simulink library "ARBI_lib"  (Simulink 7.5)
settings: Solver=ode45  StartTime=0.0  StopTime=10.0  RelTol=1e-3
values from neighbouring files (symbols this model uses):
  pARBI_st_AirbagError_C = Simulink.Parameter    [ARBI_par.m]
  pARBI_st_Crash_C = Simulink.Parameter    [ARBI_par.m]
libraries: BaseOperationLib_Browser x6, PES_CZ_FAW x2, simulink x2
settings Model: Creator=wuaibin  LastModifiedBy=wuaibin

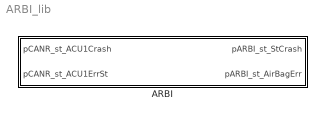
== system ARBI_lib ==
  ARBI : Subsystem  TreatAsAtomicUnit=on

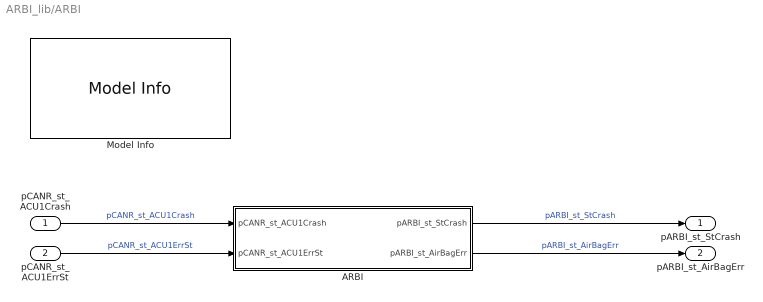
== system ARBI_lib/ARBI ==
  pCANR_st_ACU1Crash : Inport  OutDataType=fixdt(1, 16)  OutScaling=2^0
  pCANR_st_ACU1ErrSt : Inport  Port=2  OutDataType=fixdt(1, 16)  OutScaling=2^0
  ARBI : Subsystem  TreatAsAtomicUnit=on
  Model Info : simulink/Model-Wide Utilities/Model Info  SystemSampleTime=-1  InitialBlockCM=None  BlockCM=None  Frame=on  DisplayStringWithTags=Model Info\nCreated: %<Created>\nCreator: zhangqiang  HorizontalTextAlignment=Center  LeftAlignmentValue=0.5  SourceBlockDiagram=untitled  TagMaxNumber=20
  pARBI_st_StCrash : Outport  OutDataType=fixdt(1, 16)  OutScaling=2^0
  pARBI_st_AirBagErr : Outport  Port=2  OutDataType=fixdt(1, 16)  OutScaling=2^0
  wires:
  ARBI/1(pARBI_st_StCrash) -> pARBI_st_StCrash/1  "pARBI_st_StCrash"
  pCANR_st_ACU1Crash/1 -> ARBI/1(pCANR_st_ACU1Crash)  "pCANR_st_ACU1Crash"
  pCANR_st_ACU1ErrSt/1 -> ARBI/2(pCANR_st_ACU1ErrSt)  "pCANR_st_ACU1ErrSt"
  ARBI/2(pARBI_st_AirBagErr) -> pARBI_st_AirBagErr/1  "pARBI_st_AirBagErr"

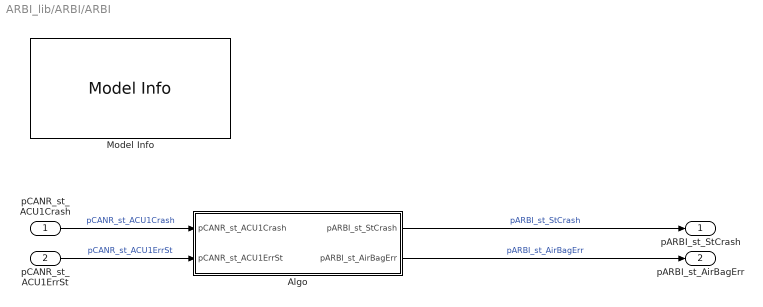
== system ARBI_lib/ARBI/ARBI ==
  pCANR_st_ACU1Crash : Inport  OutDataType=fixdt(1, 16)  OutScaling=2^0
  pCANR_st_ACU1ErrSt : Inport  Port=2  OutDataType=fixdt(1, 16)  OutScaling=2^0
  Algo : Subsystem
  Model Info : simulink/Model-Wide Utilities/Model Info  SystemSampleTime=-1  InitialBlockCM=None  BlockCM=None  Frame=on  DisplayStringWithTags=Model Info\nCreated: %<Created>\nCreator: %<Creator>  HorizontalTextAlignment=Center  LeftAlignmentValue=0.5  SourceBlockDiagram=HQEV_HCU  TagMaxNumber=20
  pARBI_st_StCrash : Outport  OutDataType=fixdt(1, 16)  OutScaling=2^0
  pARBI_st_AirBagErr : Outport  Port=2  OutDataType=fixdt(1, 16)  OutScaling=2^0
  wires:
  Algo/2(pARBI_st_AirBagErr) -> pARBI_st_AirBagErr/1  "pARBI_st_AirBagErr"
  pCANR_st_ACU1ErrSt/1 -> Algo/2(pCANR_st_ACU1ErrSt)  "pCANR_st_ACU1ErrSt"
  pCANR_st_ACU1Crash/1 -> Algo/1(pCANR_st_ACU1Crash)  "pCANR_st_ACU1Crash"
  Algo/1(pARBI_st_StCrash) -> pARBI_st_StCrash/1  "pARBI_st_StCrash"

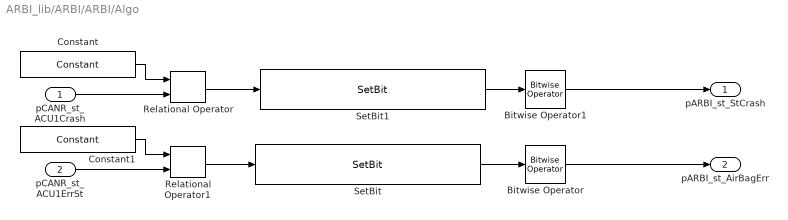
== system ARBI_lib/ARBI/ARBI/Algo ==
  pCANR_st_ACU1Crash : Inport  OutDataType=fixdt(1, 16)  OutScaling=2^0
  pCANR_st_ACU1ErrSt : Inport  Port=2  OutDataType=fixdt(1, 16)  OutScaling=2^0
  Bitwise Operator : BaseOperationLib_Browser/Others Unchanged/Bitwise Operator  logicop=OR  UseBitMask=off  BitMask=bin2dec('11011001')  BitMaskRealWorld=Stored Integer
  Bitwise Operator1 : BaseOperationLib_Browser/Others Unchanged/Bitwise Operator  logicop=OR  UseBitMask=off  BitMask=bin2dec('11011001')  BitMaskRealWorld=Stored Integer
  Constant : BaseOperationLib_Browser/Sources&Sinks/Constant  Value=pARBI_st_Crash_C  OutMin=[]  OutMax=[]  OutDataType=fixdt(1, 16)  ConRadixGroup=Use specified scaling  OutScaling=2^0  OutDataTypeStr=Inherit: Inherit from 'Constant value'
  Constant1 : BaseOperationLib_Browser/Sources&Sinks/Constant  Value=pARBI_st_AirbagError_C  OutMin=[]  OutMax=[]  OutDataType=fixdt(1, 16)  ConRadixGroup=Use specified scaling  OutScaling=2^0  OutDataTypeStr=Inherit: Inherit from 'Constant value'
  Relational Operator : BaseOperationLib_Browser/Logic Operations Changed/Relational Operator  Operator===  InputSameDT=on  LogicOutDataTypeMode=Specify via dialog  LogicDataType=PDT_Bool  OutDataTypeStr=PDT_Bool
  Relational Operator1 : BaseOperationLib_Browser/Logic Operations Changed/Relational Operator  Operator===  InputSameDT=on  LogicOutDataTypeMode=Specify via dialog  LogicDataType=PDT_Bool  OutDataTypeStr=PDT_Bool
  SetBit : PES_CZ_FAW/Discontinuities/SetBit  SystemSampleTime=-1  maska=FAWAirBagErrTyp.AIRBAG_ERROR
  SetBit1 : PES_CZ_FAW/Discontinuities/SetBit  SystemSampleTime=-1  maska=StaCrashTyp.CRASH
  pARBI_st_StCrash : Outport  OutDataType=fixdt(1, 16)  OutScaling=2^0
  pARBI_st_AirBagErr : Outport  Port=2  OutDataType=fixdt(1, 16)  OutScaling=2^0
  wires:
  SetBit1/1 -> Bitwise Operator1/1
  Bitwise Operator/1 -> pARBI_st_AirBagErr/1
  SetBit/1 -> Bitwise Operator/1
  Bitwise Operator1/1 -> pARBI_st_StCrash/1
  Relational Operator/1 -> SetBit1/1
  Relational Operator1/1 -> SetBit/1
  pCANR_st_ACU1ErrSt/1 -> Relational Operator1/2
  pCANR_st_ACU1Crash/1 -> Relational Operator/2
  Constant/1 -> Relational Operator/1
  Constant1/1 -> Relational Operator1/1
